simulink model "link_modelling"  (R2024b)
settings: Solver=FixedStepAuto  StartTime=0.0  StopTime=18  FixedStep=0.001  MaxStep=0.011111797024507685  RelTol=1e-3
values from neighbouring files (symbols this model uses):
  c_welle = 5    [flex_welle_init.m]    (also in star_welle_init.m = 900)
  d_welle = 0.1    [flex_welle_init.m]    (also in star_welle_init.m)
  thetaA = 1    [flex_welle_init.m]    (also in star_welle_init.m)
  thetaM = 0.1    [flex_welle_init.m]    (also in motor_init.m; star_welle_init.m)
settings Model: Creator=aviehweider  LastModifiedBy=aviehweider
settings RTWCC: GPUComputeCapability=3.5

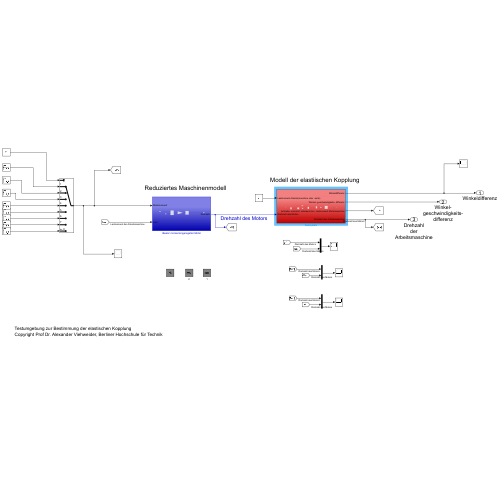
[thumbnail: Simulink's stored preview of the top-level diagram]
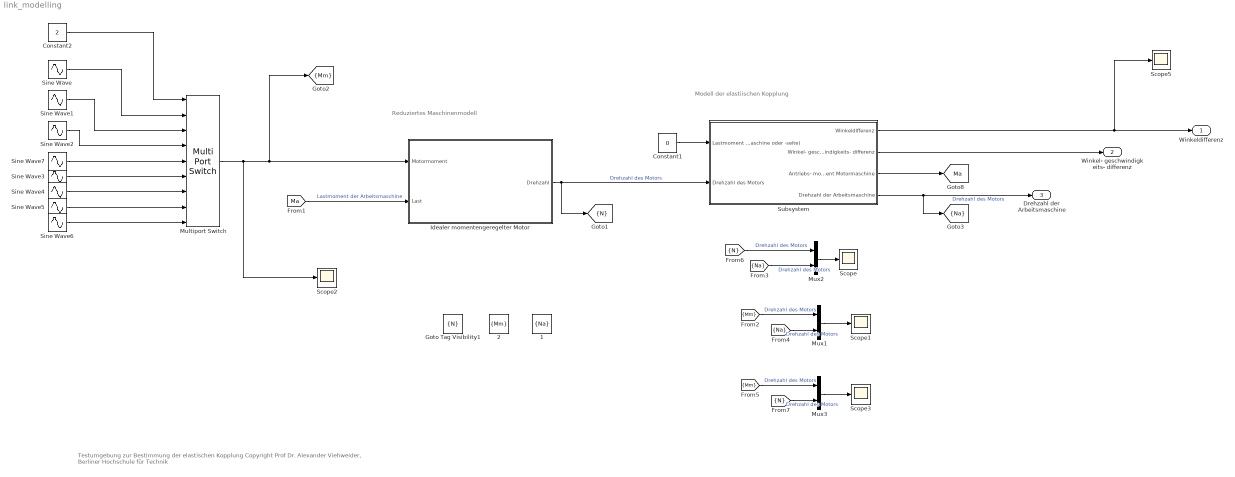
== system link_modelling ==
  note: Modell der elastiischen Kopplung
  note: Reduziertes Maschinenmodell
  note: Testumgebung zur Bestimmung der elastischen Kopplung
      | Copyright Prof Dr. Alexander Viehweider, Berliner Hochschule für Technik
  1 : GotoTagVisibility  GotoTag=Na
  2 : GotoTagVisibility  GotoTag=Mm
  Constant1 : Constant  Value=0
  Constant2 : Constant  Value=2
  Goto Tag Visibility1 : GotoTagVisibility  GotoTag=N
  Idealer momentengeregelter Motor : Subsystem
  Multiport Switch : MultiPortSwitch  Inputs=8  SaturateOnIntegerOverflow=off  InputSameDT=off
  Mux1 : Mux  Inputs=2
  Mux2 : Mux  Inputs=2
  Mux3 : Mux  Inputs=2
  Scope{,1..3,5} (5 alike) : Scope
  Sine Wave : Sin  Frequency=0.1*(2*pi)  SampleTime=0
  Sine Wave1 : Sin  Frequency=1*(2*pi)  SampleTime=0
  Sine Wave2 : Sin  Frequency=2*(2*pi)  SampleTime=0
  Sine Wave3 : Sin  Frequency=10*2*pi  SampleTime=0
  Sine Wave4 : Sin  Frequency=15.8568*2*pi  SampleTime=0
  Sine Wave5 : Sin  Frequency=20*2*pi  SampleTime=0
  Sine Wave6 : Sin  Frequency=30*2*pi  SampleTime=0
  Sine Wave7 : Sin  Frequency=5*(2*pi)  SampleTime=0
  Subsystem : Subsystem
  Winkeldifferenz : Outport
  Winkel- geschwindigkeits- differenz : Outport  Port=2
  Drehzahl der Arbeitsmaschine : Outport  Port=3
  tag scope: Ma=global, Mm=scoped, N=scoped, Na=scoped
  wires:
  Idealer momentengeregelter Motor/1(Drehzahl) -> [N], Subsystem/2(Drehzahl des Motors)  "Drehzahl des Motors"
  Subsystem/3(Antriebs- moment Lastmaschine= Lastmoment Motormaschine) -> [Ma]
  Subsystem/1(Winkeldifferenz) -> Scope5/1, Winkeldifferenz/1
  Subsystem/2(Winkel- geschwindigkeits- differenz) -> Winkel- geschwindigkeits- differenz/1
  Constant1/1 -> Subsystem/1(Lastmoment Arbeits(maschine oder -seite))
  Multiport Switch/1 -> Scope2/1, [Mm], Idealer momentengeregelter Motor/1(Motormoment)
  [Ma] -> Idealer momentengeregelter Motor/2(Last)  "Lastmoment der Arbeitsmaschine"
  Constant2/1 -> Multiport Switch/1
  [N] -> Mux2/1  "Drehzahl des Motors"
  Sine Wave6/1 -> Multiport Switch/9
  Sine Wave5/1 -> Multiport Switch/8
  Sine Wave4/1 -> Multiport Switch/7
  Sine Wave3/1 -> Multiport Switch/6
  Sine Wave/1 -> Multiport Switch/2
  Sine Wave1/1 -> Multiport Switch/3
  Sine Wave2/1 -> Multiport Switch/4
  Sine Wave7/1 -> Multiport Switch/5
  Mux2/1 -> Scope/1
  [Mm] -> Mux1/1  "Drehzahl des Motors"
  Subsystem/4(Drehzahl der Arbeitsmaschine) -> [Na], Drehzahl der Arbeitsmaschine/1  "Drehzahl des Motors"
  Mux1/1 -> Scope1/1
  [Na] -> Mux2/2  "Drehzahl des Motors"
  [Na] -> Mux1/2  "Drehzahl des Motors"
  [Mm] -> Mux3/1  "Drehzahl des Motors"
  Mux3/1 -> Scope3/1
  [N] -> Mux3/2  "Drehzahl des Motors"

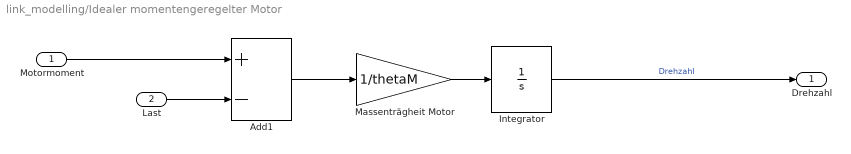
== system link_modelling/Idealer momentengeregelter Motor ==
  Motormoment : Inport
  Last : Inport  Port=2
  Add1 : Sum  Inputs=+-
  Integrator : Integrator
  Massenträgheit Motor : Gain  Gain=1/thetaM
  Drehzahl : Outport
  wires:
  Motormoment/1 -> Add1/1
  Massenträgheit Motor/1 -> Integrator/1
  Add1/1 -> Massenträgheit Motor/1
  Last/1 -> Add1/2
  Integrator/1 -> Drehzahl/1  "Drehzahl"

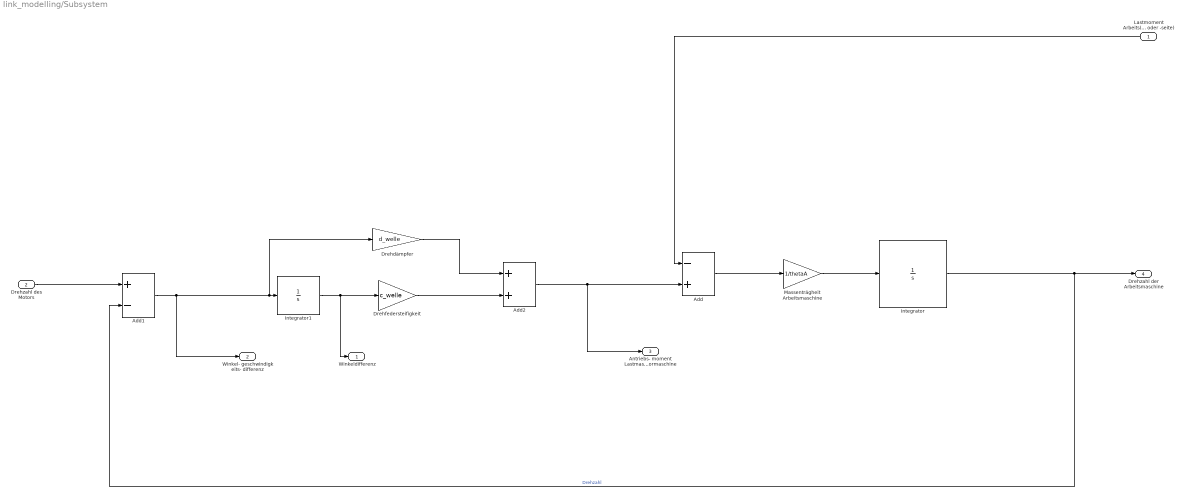
== system link_modelling/Subsystem ==
  Lastmoment Arbeits(maschine oder -seite) : Inport
  Drehzahl des Motors : Inport  Port=2
  Add : Sum  Inputs=-+
  Add1 : Sum  Inputs=+-
  Add2 : Sum
  Drehdämpfer : Gain  Gain=d_welle
  Drehfedersteifigkeit : Gain  Gain=c_welle
  Integrator : Integrator
  Integrator1 : Integrator
  Massenträgheit Arbeitsmaschine : Gain  Gain=1/thetaA
  Winkeldifferenz : Outport
  Winkel- geschwindigkeits- differenz : Outport  Port=2
  Antriebs- moment Lastmaschine= Lastmoment Motormaschine : Outport  Port=3
  Drehzahl der Arbeitsmaschine : Outport  Port=4
  wires:
  Add2/1 -> Antriebs- moment Lastmaschine= Lastmoment Motormaschine/1, Add/2
  Add1/1 -> Winkel- geschwindigkeits- differenz/1, Drehdämpfer/1, Integrator1/1
  Integrator/1 -> Drehzahl der Arbeitsmaschine/1, Add1/2  "Drehzahl"
  Drehfedersteifigkeit/1 -> Add2/2
  Massenträgheit Arbeitsmaschine/1 -> Integrator/1
  Drehdämpfer/1 -> Add2/1
  Integrator1/1 -> Winkeldifferenz/1, Drehfedersteifigkeit/1
  Add/1 -> Massenträgheit Arbeitsmaschine/1
  Drehzahl des Motors/1 -> Add1/1
  Lastmoment Arbeits(maschine oder -seite)/1 -> Add/1
